simulink model "STM32_UART_PWM_OUTPUT"  (R2024b)
settings: Solver=ode4  StartTime=0.0  StopTime=Tsim  FixedStep=0.005  RelTol=1e-3  EnableMultiTasking=on
values from neighbouring files (symbols this model uses):
  circle_dir = 1    [STM32_UART_PWM_OUTPUT_SETUP.m]
  DEG_TO_RAD_F32 = single(pi / 180.0)    [STM32_UART_PWM_OUTPUT_SETUP.m]
  delta_corr_max_rad = single(deg2rad(8.0))    [STM32_UART_PWM_OUTPUT_SETUP.m]
  delta_max_rad = deg2rad(25)    [STM32_UART_PWM_OUTPUT_SETUP.m]
  delta_test_rad = deg2rad(14.6)    [STM32_UART_PWM_OUTPUT_SETUP.m]
  Kd_psi_pid = single(0.0)    [STM32_UART_PWM_OUTPUT_SETUP.m]
  Kd_radius_pid = single(0.0)    [STM32_UART_PWM_OUTPUT_SETUP.m]
  Ki_psi_pid = single(0.0)    [STM32_UART_PWM_OUTPUT_SETUP.m]
  Ki_radius_pid = single(0.0)    [STM32_UART_PWM_OUTPUT_SETUP.m]
  Kp_psi_pid = single(1.0)    [STM32_UART_PWM_OUTPUT_SETUP.m]
  Kp_radius_pid = single(0.65)    [STM32_UART_PWM_OUTPUT_SETUP.m]
  L = 0.26    [STM32_UART_PWM_OUTPUT_SETUP.m]
  psi_offset_max_rad = single(deg2rad(18.0))    [STM32_UART_PWM_OUTPUT_SETUP.m]
  R_ref = 1.0    (= 1)    [STM32_UART_PWM_OUTPUT_SETUP.m]
  Ts_base = 0.005    [STM32_UART_PWM_OUTPUT_SETUP.m]
  xc = 0.0    (= 0)    [STM32_UART_PWM_OUTPUT_SETUP.m]
  yc = 0.0    (= 0)    [STM32_UART_PWM_OUTPUT_SETUP.m]
libraries: slpidlib x2, stm32f4xxblockslib x1, stm32blockslib x1
settings Model: STM32="{\"UARTRead\":{\"ID\":\"STM32_UART_PWM_OUTPUT:145\"},\"PWMOutput\":{\"ID\":\"STM32_UART_PWM_OUTPUT:160\"}}"  Creator=mateu  LastModifiedBy=mateu
settings OptimizationCC: DefaultParameterBehavior=Inlined  EnhancedBackFolding=on  PassReuseOutputArgsAs=Individual arguments  ZeroExternalMemoryAtStartup=off  ZeroInternalMemoryAtStartup=off  MaxStackSize=512  OptimizeBlockOrder=speed  DifferentSizesBufferReuse=on  OptimizationCustomize=off  EfficientTunableParamExpr=on
settings DebuggingCC: ParameterTunabilityLossMsg=error
settings HardwareCC: ProdBitPerPointer=32  ProdBitPerSizeT=32  ProdBitPerPtrDiffT=32  ProdLargestAtomicInteger=Long  ProdLargestAtomicFloat=Double  ProdWordSize=32  ProdLongLongMode=on  ProdHWDeviceType=ARM Compatible->ARM Cortex-M
settings SFSimCC: MATLABDynamicMemAlloc=off
settings RTWCC: Description=Embedded Coder  SystemTargetFile=ert.tlc  HardwareBoard=STM32L4xx Based  TemplateMakefile=ert_default_tmf  Toolchain=GNU Tools for ARM Embedded Processors
settings CodeAppCC: ForceParamTrailComments=on  IgnoreCustomStorageClasses=off  OperatorAnnotations=on  SimulinkDataObjDesc=on  SFDataObjDesc=on  InsertBlockDesc=on
settings ERTTargetCC: TargetLangStandard=C99 (ISO)  CodeReplacementLibrary=ARM Cortex-M  ExtModeTransport=3  ExtModeStaticAlloc=on  ExtModeStaticAllocSize=2048  ExtModeMexFile=ext_xcp  ExtModeIntrfLevel=Level2 - Open

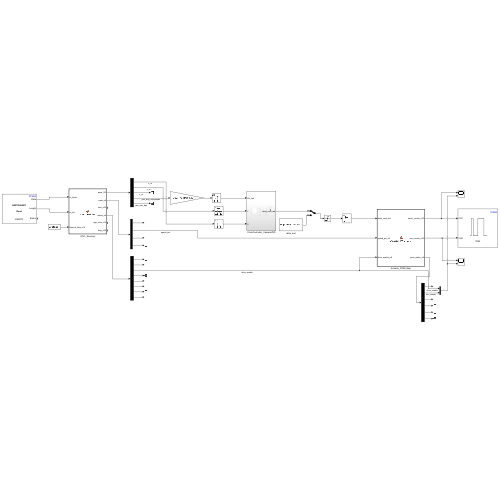
[thumbnail: Simulink's stored preview of the top-level diagram]
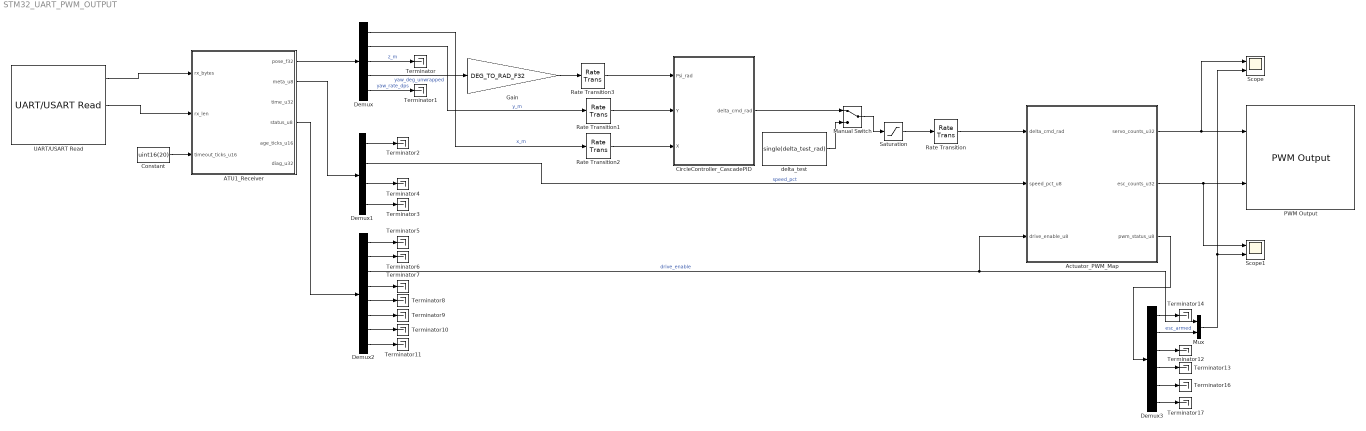
== system STM32_UART_PWM_OUTPUT ==
  ATU1_Receiver : MATLAB Function  TreatAsAtomicUnit=on
  Actuator_PWM_Map : MATLAB Function  TreatAsAtomicUnit=on
  CircleController_CascadePID : Subsystem
  Constant : Constant  Value=uint16(20)
  Demux : Demux  Outputs=5
  Demux1 : Demux
  Demux2 : Demux  Outputs=8
  Demux3 : Demux  Outputs=6
  Gain : Gain  Gain=DEG_TO_RAD_F32
  Manual Switch : ManualSwitch
  Mux : Mux  Inputs=2
  PWM Output : stm32f4xxblockslib/PWM Output  TimerModule=TIM2  DutycycleUnits=Counts  EnableChannel1=on  EnableChannel2=on  EnableChannel3=off  EnableChannel4=off  EnableCounterInput=off  EnableMainOutputInput=off  EnableFrequencyInput=off  SetRCAfterCE=off  OutputDirection=off  OutputMainOutputEnableStatus=off  SampleTime=0.1  EnableSimPort=off  EnableUpdateEvent=off  EnableCaptureCompare1Event=off  EnableCaptureCompare2Event=off  EnableCaptureCompare3Event=off  EnableCaptureCompare4Event=off  EnableTriggerEvent=off  EnableBreakEvent=off  ProcessorFamily=STM32F4  hoistedMaskSrc=ECSoC/ECSimCodegen/PWM Output
  Rate Transition : RateTransition  OutPortSampleTime=Ts_base
  Rate Transition1 : RateTransition  OutPortSampleTime=Ts_control
  Rate Transition2 : RateTransition  OutPortSampleTime=Ts_control
  Rate Transition3 : RateTransition  OutPortSampleTime=Ts_control
  Saturation : Saturate  UpperLimit=delta_max_rad  LowerLimit=-delta_max_rad
  Scope : Scope  NumInputPorts=2
  Scope1 : Scope  NumInputPorts=2
  Terminator{,1..14,16..17} (17 alike) : Terminator
  UART/USART Read : stm32blockslib/UART//USART Read  UARTModule=USART3  DataType=uint8  DataLength=64  BlockingMode=off  BlockingTimeout=0.1  OutputLength=on  OutputStatus=on  SampleTime=Ts_base
      settings: LibrarySourceBlock=stm32f4xxblockslib/UART//USART Read
  delta_test : Constant  Value=single(delta_test_rad)
  wires:
  UART/USART Read/1 -> ATU1_Receiver/1(rx_bytes)
  UART/USART Read/2 -> ATU1_Receiver/2(rx_len)
  Demux/4 -> Gain/1  "yaw_deg_unwrapped"
  Rate Transition1/1 -> CircleController_CascadePID/2(Y)
  Rate Transition2/1 -> CircleController_CascadePID/1(X)
  ATU1_Receiver/1(pose_f32) -> Demux/1
  Demux/1 -> Rate Transition2/1  "x_m"
  Demux/2 -> Rate Transition1/1  "y_m"
  Demux/3 -> Terminator/1  "z_m"
  Demux/5 -> Terminator1/1  "yaw_rate_dps"
  Rate Transition3/1 -> CircleController_CascadePID/3(Psi_rad)
  Gain/1 -> Rate Transition3/1
  CircleController_CascadePID/1(delta_cmd_rad) -> Manual Switch/1
  delta_test/1 -> Manual Switch/2
  Manual Switch/1 -> Saturation/1
  Constant/1 -> ATU1_Receiver/3(timeout_ticks_u16)
  Saturation/1 -> Rate Transition/1
  ATU1_Receiver/2(meta_u8) -> Demux1/1
  Demux1/1 -> Terminator2/1
  Demux1/3 -> Terminator4/1
  Demux1/4 -> Terminator3/1
  ATU1_Receiver/4(status_u8) -> Demux2/1
  Demux2/1 -> Terminator5/1
  Demux2/2 -> Terminator6/1
  Demux2/4 -> Terminator7/1
  Demux2/5 -> Terminator8/1
  Demux2/6 -> Terminator9/1
  Demux2/7 -> Terminator10/1
  Demux2/8 -> Terminator11/1
  Rate Transition/1 -> Actuator_PWM_Map/1(delta_cmd_rad)
  Demux1/2 -> Actuator_PWM_Map/2(speed_pct_u8)  "speed_pct"
  Demux2/3 -> Mux/1, Actuator_PWM_Map/3(drive_enable_u8)  "drive_enable"
  Actuator_PWM_Map/1(servo_counts_u32) -> Scope/1, PWM Output/1
  Actuator_PWM_Map/2(esc_counts_u32) -> Scope1/1, PWM Output/2
  Actuator_PWM_Map/3(pwm_status_u8) -> Demux3/1
  Demux3/1 -> Terminator14/1
  Demux3/2 -> Mux/2  "esc_armed"
  Demux3/3 -> Terminator12/1
  Demux3/4 -> Terminator13/1
  Demux3/5 -> Terminator16/1
  Demux3/6 -> Terminator17/1
  Mux/1 -> Scope/2, Scope1/2

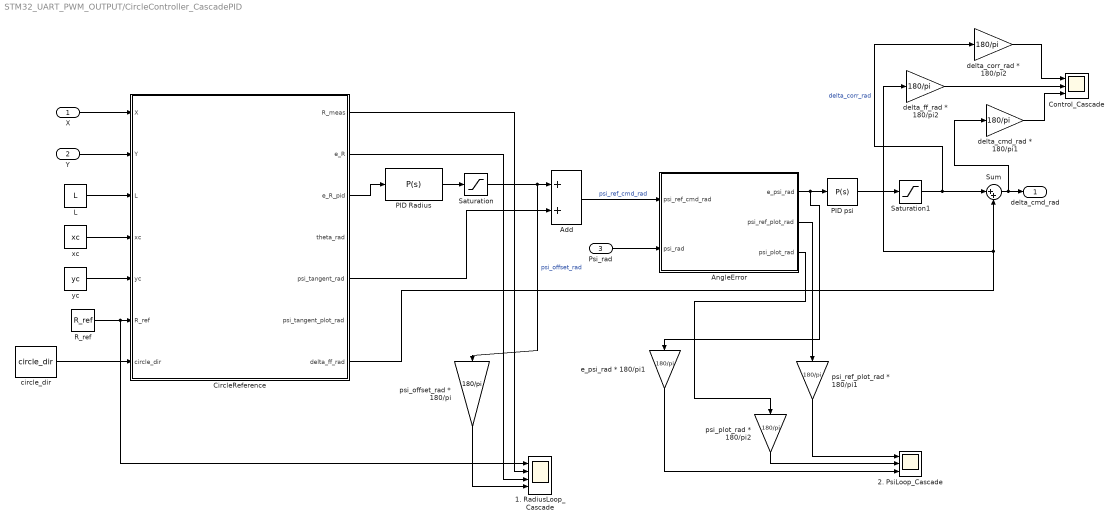
== system STM32_UART_PWM_OUTPUT/CircleController_CascadePID ==
  X : Inport
  Y : Inport  Port=2
  Psi_rad : Inport  Port=3
  1. RadiusLoop_Cascade : Scope  NumInputPorts=4
  2. PsiLoop_Cascade : Scope  NumInputPorts=3
  Add : Sum
  AngleError : MATLAB Function  TreatAsAtomicUnit=on
  CircleReference : MATLAB Function  TreatAsAtomicUnit=on
  Control_Cascade : Scope  NumInputPorts=3
  L : Constant  Value=L
  PID Radius : slpidlib/PID Controller  Controller=P  Form=Parallel  TimeDomain=Continuous-time  UseExternalTs=off  SampleTime=-1  IntegratorMethod=Forward Euler  FilterMethod=Forward Euler  ControllerParametersSource=internal  P=Kp_radius_pid  I=Ki_radius_pid  UseKiTs=off  D=Kd_radius_pid  UseExternalDerivativeSource=off  N=171.856773592637  UseFilter=on  TunerSelectOption=Transfer Function Based (PID Tuner App)  InitialConditionSource=internal  InitialConditionForIntegrator=0  InitialConditionForFilter=0  DifferentiatorICPrevScaledInput=0  ExternalReset=none  TrackingMode=off  Kt=1  LimitOutput=off  SatLimitsSource=internal  UpperSaturationLimit=inf  LowerSaturationLimit=-inf  LinearizeAsGain=on  AntiWindupMode=none  Kb=1  LimitIntegrator=off  UpperIntegratorSaturationLimit=inf  LowerIntegratorSaturationLimit=-inf  POutMin=[]  POutMax=[]  IOutMin=[]  IOutMax=[]  DOutMin=[]  DOutMax=[]  NOutMin=[]  NOutMax=[]  SumOutMin=[]  SumOutMax=[]  SaturationOutMin=[]  SaturationOutMax=[]  PParamMin=[]  PParamMax=[]  IParamMin=[]  IParamMax=[]  DParamMin=[]  DParamMax=[]  NParamMin=[]  NParamMax=[]  KbParamMin=[]  KbParamMax=[]  KtParamMin=[]  KtParamMax=[]  KbOutMin=[]  KbOutMax=[]  KtOutMin=[]  KtOutMax=[]  IntegratorOutMin=[]  IntegratorOutMax=[]  FilterOutMin=[]  FilterOutMax=[]  SumI1OutMin=[]  SumI1OutMax=[]  SumI2OutMin=[]  SumI2OutMax=[]  SumI3OutMin=[]  SumI3OutMax=[]  SumI4OutMin=[]  SumI4OutMax=[]  SumDOutMin=[]  SumDOutMax=[]  DifferentiatorOutMin=[]  DifferentiatorOutMax=[]  FilterDiffOutCoefMin=[]  FilterDiffOutCoefMax=[]  ReciprocalOutMin=[]  ReciprocalOutMax=[]  SumDenOutMin=[]  SumDenOutMax=[]  SumNumOutMin=[]  SumNumOutMax=[]  DivideOutMin=[]  DivideOutMax=[]  UdiffTsProdOutMin=[]  UdiffTsProdOutMax=[]  NTsProdOutMin=[]  NTsProdOutMax=[]  UintegralTsProdOutMin=[]  UintegralTsProdOutMax=[]  UngainTsProdOutMin=[]  UngainTsProdOutMax=[]  ClampingZeroOutDataTypeStr=Inherit: Inherit via back propagation  ClampingZeroOutMin=[]  ClampingZeroOutMax=[]  FilterDenConstantOutDataTypeStr=Inherit: Inherit via back propagation  FilterDenConstantOutMin=[]  FilterDenConstantOutMax=[]  PCopyOutDataTypeStr=Inherit: Inherit via back propagation  PCopyOutMin=[]  PCopyOutMax=[]  NCopyOutDataTypeStr=Inherit: Inherit via back propagation  NCopyOutMin=[]  NCopyOutMax=[]  IntegratorContinuousStateAttributes=''  IntegratorStateMustResolveToSignalObject=off  IntegratorRTWStateStorageClass=Auto  FilterContinuousStateAttributes=''  FilterStateMustResolveToSignalObject=off  FilterRTWStateStorageClass=Auto  ParallelPVariant=InternalParameters  IdealPVariant=Disabled  IVariant=Disabled  DVariant=Disabled  IntegratorVariant=Disabled  SatVariant=Disabled  AWVariant=Disabled  PCopyVariant=Disabled  TRVariant=Disabled  FdbkBlocksVariant=Forward  IdealPFdbkVariant=Disabled  SatFdbkVariant=Disabled  DerivativeFilterVariant=Disabled  NVariant=Disabled  NCopyVariant=Disabled_SignalSpec  FilterICVariant=Disabled  IntegratorICVariant=Disabled  ExternalResetVariant=Disabled  TRSumVariant=Passthrough  SumFdbkVariant=Disabled  SumVariant=Passthrough_P  TsampFilterVariant=InternalTs  TsampNgainVariant=Passthrough  TsampIntegralVariant=Disabled_SignalSpec  ExternalSaturationOutDataTypeStr=Inherit: Same as second input  DerivativeSourceVariant=Disabled  PreIntVariant=InternalPreInt
  PID psi : slpidlib/PID Controller  Controller=P  Form=Parallel  TimeDomain=Continuous-time  UseExternalTs=off  SampleTime=-1  IntegratorMethod=Forward Euler  FilterMethod=Forward Euler  ControllerParametersSource=internal  P=Kp_psi_pid  I=Ki_psi_pid  UseKiTs=off  D=Kd_psi_pid  UseExternalDerivativeSource=off  N=184.215923888363  UseFilter=on  TunerSelectOption=Transfer Function Based (PID Tuner App)  InitialConditionSource=internal  InitialConditionForIntegrator=0  InitialConditionForFilter=0  DifferentiatorICPrevScaledInput=0  ExternalReset=none  TrackingMode=off  Kt=1  LimitOutput=off  SatLimitsSource=internal  UpperSaturationLimit=inf  LowerSaturationLimit=-inf  LinearizeAsGain=on  AntiWindupMode=none  Kb=1  LimitIntegrator=off  UpperIntegratorSaturationLimit=inf  LowerIntegratorSaturationLimit=-inf  POutMin=[]  POutMax=[]  IOutMin=[]  IOutMax=[]  DOutMin=[]  DOutMax=[]  NOutMin=[]  NOutMax=[]  SumOutMin=[]  SumOutMax=[]  SaturationOutMin=[]  SaturationOutMax=[]  PParamMin=[]  PParamMax=[]  IParamMin=[]  IParamMax=[]  DParamMin=[]  DParamMax=[]  NParamMin=[]  NParamMax=[]  KbParamMin=[]  KbParamMax=[]  KtParamMin=[]  KtParamMax=[]  KbOutMin=[]  KbOutMax=[]  KtOutMin=[]  KtOutMax=[]  IntegratorOutMin=[]  IntegratorOutMax=[]  FilterOutMin=[]  FilterOutMax=[]  SumI1OutMin=[]  SumI1OutMax=[]  SumI2OutMin=[]  SumI2OutMax=[]  SumI3OutMin=[]  SumI3OutMax=[]  SumI4OutMin=[]  SumI4OutMax=[]  SumDOutMin=[]  SumDOutMax=[]  DifferentiatorOutMin=[]  DifferentiatorOutMax=[]  FilterDiffOutCoefMin=[]  FilterDiffOutCoefMax=[]  ReciprocalOutMin=[]  ReciprocalOutMax=[]  SumDenOutMin=[]  SumDenOutMax=[]  SumNumOutMin=[]  SumNumOutMax=[]  DivideOutMin=[]  DivideOutMax=[]  UdiffTsProdOutMin=[]  UdiffTsProdOutMax=[]  NTsProdOutMin=[]  NTsProdOutMax=[]  UintegralTsProdOutMin=[]  UintegralTsProdOutMax=[]  UngainTsProdOutMin=[]  UngainTsProdOutMax=[]  ClampingZeroOutDataTypeStr=Inherit: Inherit via back propagation  ClampingZeroOutMin=[]  ClampingZeroOutMax=[]  FilterDenConstantOutDataTypeStr=Inherit: Inherit via back propagation  FilterDenConstantOutMin=[]  FilterDenConstantOutMax=[]  PCopyOutDataTypeStr=Inherit: Inherit via back propagation  PCopyOutMin=[]  PCopyOutMax=[]  NCopyOutDataTypeStr=Inherit: Inherit via back propagation  NCopyOutMin=[]  NCopyOutMax=[]  IntegratorContinuousStateAttributes=''  IntegratorStateMustResolveToSignalObject=off  IntegratorRTWStateStorageClass=Auto  FilterContinuousStateAttributes=''  FilterStateMustResolveToSignalObject=off  FilterRTWStateStorageClass=Auto  ParallelPVariant=InternalParameters  IdealPVariant=Disabled  IVariant=Disabled  DVariant=Disabled  IntegratorVariant=Disabled  SatVariant=Disabled  AWVariant=Disabled  PCopyVariant=Disabled  TRVariant=Disabled  FdbkBlocksVariant=Forward  IdealPFdbkVariant=Disabled  SatFdbkVariant=Disabled  DerivativeFilterVariant=Disabled  NVariant=Disabled  NCopyVariant=Disabled_SignalSpec  FilterICVariant=Disabled  IntegratorICVariant=Disabled  ExternalResetVariant=Disabled  TRSumVariant=Passthrough  SumFdbkVariant=Disabled  SumVariant=Passthrough_P  TsampFilterVariant=InternalTs  TsampNgainVariant=Passthrough  TsampIntegralVariant=Disabled_SignalSpec  ExternalSaturationOutDataTypeStr=Inherit: Same as second input  DerivativeSourceVariant=Disabled  PreIntVariant=InternalPreInt
  R_ref : Constant  Value=R_ref
  Saturation : Saturate  UpperLimit=psi_offset_max_rad  LowerLimit=-psi_offset_max_rad
  Saturation1 : Saturate  UpperLimit=delta_corr_max_rad  LowerLimit=-delta_corr_max_rad
  Sum : Sum  Inputs=|++
  circle_dir : Constant  Value=circle_dir
  delta_cmd_rad * 180/pi1 : Gain  Gain=180/pi
  delta_corr_rad * 180/pi2 : Gain  Gain=180/pi
  delta_ff_rad * 180/pi2 : Gain  Gain=180/pi
  e_psi_rad * 180/pi1 : Gain  Gain=180/pi
  psi_offset_rad * 180/pi : Gain  Gain=180/pi
  psi_plot_rad * 180/pi2 : Gain  Gain=180/pi
  psi_ref_plot_rad * 180/pi1 : Gain  Gain=180/pi
  xc : Constant  Value=xc
  yc : Constant  Value=yc
  delta_cmd_rad : Outport
  wires:
  X/1 -> CircleReference/1(X)
  Y/1 -> CircleReference/2(Y)
  yc/1 -> CircleReference/5(yc)
  R_ref/1 -> 1. RadiusLoop_Cascade/1, CircleReference/6(R_ref)
  circle_dir/1 -> CircleReference/7(circle_dir)
  L/1 -> CircleReference/3(L)
  xc/1 -> CircleReference/4(xc)
  CircleReference/3(e_R_pid) -> PID Radius/1
  PID Radius/1 -> Saturation/1
  Saturation/1 -> psi_offset_rad * 180/pi/1, Add/1  "psi_offset_rad"
  CircleReference/5(psi_tangent_rad) -> Add/2
  Add/1 -> AngleError/1(psi_ref_cmd_rad)  "psi_ref_cmd_rad"
  Psi_rad/1 -> AngleError/2(psi_rad)
  PID psi/1 -> Saturation1/1
  Saturation1/1 -> delta_corr_rad * 180/pi2/1, Sum/1  "delta_corr_rad"
  Sum/1 -> delta_cmd_rad * 180/pi1/1, delta_cmd_rad/1
  CircleReference/7(delta_ff_rad) -> delta_ff_rad * 180/pi2/1, Sum/2
  CircleReference/1(R_meas) -> 1. RadiusLoop_Cascade/2
  CircleReference/2(e_R) -> 1. RadiusLoop_Cascade/3
  psi_offset_rad * 180/pi/1 -> 1. RadiusLoop_Cascade/4
  AngleError/2(psi_ref_plot_rad) -> psi_ref_plot_rad * 180/pi1/1
  psi_ref_plot_rad * 180/pi1/1 -> 2. PsiLoop_Cascade/1
  psi_plot_rad * 180/pi2/1 -> 2. PsiLoop_Cascade/2
  e_psi_rad * 180/pi1/1 -> 2. PsiLoop_Cascade/3
  AngleError/3(psi_plot_rad) -> psi_plot_rad * 180/pi2/1
  delta_corr_rad * 180/pi2/1 -> Control_Cascade/1
  delta_ff_rad * 180/pi2/1 -> Control_Cascade/2
  delta_cmd_rad * 180/pi1/1 -> Control_Cascade/3
  AngleError/1(e_psi_rad) -> e_psi_rad * 180/pi1/1, PID psi/1

== matlab function STM32_UART_PWM_OUTPUT/Actuator_PWM_Map ==
  data: delta_cmd_rad input; servo_counts_u32 output; speed_pct_u8 input; drive_enable_u8 input; esc_counts_u32 output; pwm_status_u8 output
function [servo_counts_u32, esc_counts_u32, pwm_status_u8] = ...
    Actuator_PWM_Map(delta_cmd_rad, speed_pct_u8, drive_enable_u8)
%#codegen
%
% =========================================================
% Actuator_PWM_Map
% =========================================================
%
% Zamienia:
%   delta_cmd_rad  → impuls serwa TIM2_CH1
%   speed_pct      → impuls ESC TIM2_CH2
%
% Konfiguracja TIM2 w CubeMX:
%   timer clock po prescalerze = 1 MHz
%   1 count = 1 us
%   ARR = 19999
%   okres = 20 ms = 50 Hz
%
% Wejścia:
%   delta_cmd_rad    single  - zadany kąt skrętu [rad]
%   speed_pct_u8     uint8   - komenda 0...100%
%   drive_enable_u8  uint8   - zezwolenie STM32
%
% Wyjścia:
%   servo_counts_u32 uint32  - CCR dla TIM2_CH1
%   esc_counts_u32   uint32  - CCR dla TIM2_CH2
%
% pwm_status_u8:
%   1 = wejściowe drive_enable
%   2 = ESC uzbrojony
%   3 = końcowe actuator_enable
%   4 = skręt ograniczony
%   5 = prędkość ograniczona
%   6 = speed_pct po ograniczeniu
% =========================================================

% ---------------------------------------------------------
% Parametry serwa
% ---------------------------------------------------------

SERVO_LEFT_US   = single(1300.0);
SERVO_CENTER_US = single(1500.0);
SERVO_RIGHT_US  = single(1700.0);

% Początkowy bezpieczny zakres skrętu: +/-10 stopni
SERVO_DELTA_MAX_RAD = single(10.0 * pi / 180.0);

% Zmień na -1, jeżeli serwo skręca odwrotnie
SERVO_DIRECTION = single(1.0);

% ---------------------------------------------------------
% Parametry ESC
% ---------------------------------------------------------

ESC_NEUTRAL_US     = single(1500.0);
ESC_FORWARD_MAX_US = single(2000.0);

% Początkowo maksymalnie 10% komendy
SPEED_TEST_MAX_PCT = single(10.0);

% Ts_base = 0.005 s
% 600 kroków * 0.005 s = 3 sekundy neutralnego sygnału
ESC_ARM_TICKS = uint16(600);

% ---------------------------------------------------------
% Stan uzbrajania ESC
% ---------------------------------------------------------

persistent arm_counter_u16

if isempty(arm_counter_u16)
    arm_counter_u16 = uint16(0);
end

if arm_counter_u16 < ESC_ARM_TICKS
    arm_counter_u16 = arm_counter_u16 + uint16(1);
end

esc_armed = arm_counter_u16 >= ESC_ARM_TICKS;

drive_enable = drive_enable_u8 ~= uint8(0);

actuator_enable = ...
    drive_enable && ...
    esc_armed;

% =========================================================
% SERWO
% =========================================================

delta_requested_rad = single(delta_cmd_rad);

delta_limited_rad = min( ...
    max(delta_requested_rad, -SERVO_DELTA_MAX_RAD), ...
    SERVO_DELTA_MAX_RAD);

steering_limited = ...
    delta_requested_rad ~= delta_limited_rad;

delta_servo_rad = ...
    SERVO_DIRECTION * delta_limited_rad;

delta_normalized = ...
    delta_servo_rad / SERVO_DELTA_MAX_RAD;

if delta_normalized >= single(0.0)

    % 0...+1:
    % środek → prawa strona
    servo_pulse_us = ...
        SERVO_CENTER_US + ...
        delta_normalized * ...
        (SERVO_RIGHT_US - SERVO_CENTER_US);

else

    % -1...0:
    % lewa strona → środek
    servo_pulse_us = ...
        SERVO_CENTER_US + ...
        delta_normalized * ...
        (SERVO_CENTER_US - SERVO_LEFT_US);

end

% Bez zezwolenia serwo wraca na środek
if ~actuator_enable
    servo_pulse_us = SERVO_CENTER_US;
end

servo_pulse_us = min( ...
    max(servo_pulse_us, SERVO_LEFT_US), ...
    SERVO_RIGHT_US);

% =========================================================
% ESC
% =========================================================

speed_requested_pct = single(speed_pct_u8);

% Ograniczenie pełnego zakresu wejściowego
speed_requested_pct = min( ...
    max(speed_requested_pct, single(0.0)), ...
    single(100.0));

% Dodatkowe ograniczenie pierwszych testów
speed_limited_pct = min( ...
    speed_requested_pct, ...
    SPEED_TEST_MAX_PCT);

speed_limited = ...
    speed_requested_pct ~= speed_limited_pct;

% 0% → 1500 us
% 100% → 2000 us
% Przy limicie 10% maksymalny impuls wyniesie 1550 us
esc_pulse_us = ...
    ESC_NEUTRAL_US + ...
    (speed_limited_pct / single(100.0)) * ...
    (ESC_FORWARD_MAX_US - ESC_NEUTRAL_US);

% Brak zezwolenia lub uzbrajanie → neutral
if ~actuator_enable
    esc_pulse_us = ESC_NEUTRAL_US;
end

esc_pulse_us = min( ...
    max(esc_pulse_us, ESC_NEUTRAL_US), ...
    ESC_FORWARD_MAX_US);

% =========================================================
% Wyjścia TIM2 CCR
% =========================================================

servo_counts_u32 = uint32(round(servo_pulse_us));
esc_counts_u32   = uint32(round(esc_pulse_us));

pwm_status_u8 = zeros(6, 1, 'uint8');

pwm_status_u8(1) = uint8(drive_enable);
pwm_status_u8(2) = uint8(esc_armed);
pwm_status_u8(3) = uint8(actuator_enable);
pwm_status_u8(4) = uint8(steering_limited);
pwm_status_u8(5) = uint8(speed_limited);
pwm_status_u8(6) = uint8(round(speed_limited_pct));

end

== matlab function STM32_UART_PWM_OUTPUT/ATU1_Receiver ==
  data: rx_bytes input; pose_f32 output; rx_len input; meta_u8 output; time_u32 output; status_u8 output; age_ticks_u16 output; diag_u32 output; timeout_ticks_u16 input
function [pose_f32, meta_u8, time_u32, status_u8, ...
          age_ticks_u16, diag_u32] = ...
    ATU1_Receiver(rx_bytes, rx_len, timeout_ticks_u16)

% =========================================================
% ATU1_Receiver
% =========================================================
%
% Wejścia:
%
%   rx_bytes [64x1] uint8
%       bajty odebrane z UART/USART Read
%
%   rx_len [1x1] uint8
%       rzeczywista liczba nowych bajtów
%
% Wyjścia:
%
%   pose_f32 [5x1] single
%       1 = x_m
%       2 = y_m
%       3 = z_m
%       4 = yaw_deg_unwrapped
%       5 = yaw_rate_dps
%
%   meta_u8 [4x1] uint8
%       1 = flags
%       2 = speed_pct
%       3 = fps_hz
%       4 = source_id
%
%   time_u32 [2x1] uint32
%       1 = seq
%       2 = unity_t_ms
%
%   status_u8 [8x1] uint8
%       1 = new_frame
%       2 = frame_fresh
%       3 = drive_enable
%       4 = pose_valid
%       5 = deadman
%       6 = move_en
%       7 = safe_to_drive
%       8 = hard_stop
%
%   age_ticks_u16
%       liczba kroków modelu od ostatniej poprawnej ramki
%
%   diag_u32 [4x1] uint32
%       1 = frames_ok
%       2 = crc_bad
%       3 = format_bad
%       4 = timeout_count
%
% Ramka ATU1:
%
%   1-2   header A5 5A
%   3     version 1
%   4     source_id
%   5-8   seq uint32 LE
%   9-12  unity_t_ms uint32 LE
%   13    flags
%   14    speed_pct
%   15    fps_hz
%   16    reserved
%   17-20 x_m single LE
%   21-24 y_m single LE
%   25-28 z_m single LE
%   29-32 yaw_deg_unwrapped single LE
%   33-36 yaw_rate_dps single LE
%   37-38 CRC16 CCITT-FALSE LE
%
% =========================================================

persistent frame_buffer
persistent frame_count

persistent last_pose
persistent last_meta
persistent last_time

persistent age_ticks
persistent frame_seen
persistent previous_frame_fresh

persistent frames_ok
persistent crc_bad
persistent format_bad
persistent timeout_count

if isempty(frame_count)

    frame_buffer = zeros(38, 1, 'uint8');
    frame_count = uint8(0);

    last_pose = zeros(5, 1, 'single');
    last_meta = zeros(4, 1, 'uint8');
    last_time = zeros(2, 1, 'uint32');

    age_ticks = uint16(65535);
    frame_seen = false;
    previous_frame_fresh = false;

    frames_ok = uint32(0);
    crc_bad = uint32(0);
    format_bad = uint32(0);
    timeout_count = uint32(0);
end

new_frame = false;

% =========================================================
% Liczenie wieku ostatniej poprawnej ramki
% =========================================================

if frame_seen

    if age_ticks < uint16(65535)
        age_ticks = age_ticks + uint16(1);
    end

end

% Ograniczenie długości do rozmiaru wejścia
number_of_bytes = uint16(rx_len(1));

if number_of_bytes > uint16(64)
    number_of_bytes = uint16(64);
end

% =========================================================
% Parser strumienia UART
% =========================================================

for k = 1:64

    if uint16(k) <= number_of_bytes

        current_byte = rx_bytes(k);

        % -------------------------------------------------
        % Szukanie pierwszego bajtu nagłówka: 0xA5
        % -------------------------------------------------

        if frame_count == uint8(0)

            if current_byte == uint8(165)

                frame_buffer(1) = current_byte;
                frame_count = uint8(1);

            end

        % -------------------------------------------------
        % Szukanie drugiego bajtu nagłówka: 0x5A
        % -------------------------------------------------

        elseif frame_count == uint8(1)

            if current_byte == uint8(90)

                frame_buffer(2) = current_byte;
                frame_count = uint8(2);

            elseif current_byte == uint8(165)

                % Kolejny 0xA5 może być początkiem nagłówka
                frame_buffer(1) = current_byte;
                frame_count = uint8(1);

            else

                frame_count = uint8(0);

            end

        % -------------------------------------------------
        % Zbieranie pozostałych bajtów
        % -------------------------------------------------

        else

            write_index = double(frame_count) + 1.0;

            frame_buffer(write_index) = current_byte;
            frame_count = frame_count + uint8(1);

            % ---------------------------------------------
            % Odebrano kompletne 38 bajtów
            % ---------------------------------------------

            if frame_count == uint8(38)

                header_ok = ...
                    frame_buffer(1) == uint8(165) && ...
                    frame_buffer(2) == uint8(90);

                version_ok = ...
                    frame_buffer(3) == uint8(1);

                received_crc = bitor( ...
                    uint16(frame_buffer(37)), ...
                    bitshift(uint16(frame_buffer(38)), 8) ...
                );

                calculated_crc = ...
                    crc16_ccitt_false_36bytes(frame_buffer);

                if header_ok && version_ok && ...
                        received_crc == calculated_crc

                    % -------------------------------------
                    % Meta
                    % -------------------------------------

                    last_meta(1) = frame_buffer(13); % flags
                    last_meta(2) = frame_buffer(14); % speed
                    last_meta(3) = frame_buffer(15); % fps
                    last_meta(4) = frame_buffer(4);  % source

                    % -------------------------------------
                    % Czasy
                    % -------------------------------------

                    last_time(1) = ...
                        read_u32_le(frame_buffer, 5);

                    last_time(2) = ...
                        read_u32_le(frame_buffer, 9);

                    % -------------------------------------
                    % Pozycja
                    % -------------------------------------

                    last_pose(1) = ...
                        read_f32_le(frame_buffer, 17);

                    last_pose(2) = ...
                        read_f32_le(frame_buffer, 21);

                    last_pose(3) = ...
                        read_f32_le(frame_buffer, 25);

                    last_pose(4) = ...
                        read_f32_le(frame_buffer, 29);

                    last_pose(5) = ...
                        read_f32_le(frame_buffer, 33);

                    frames_ok = frames_ok + uint32(1);

                    new_frame = true;
                    frame_seen = true;
                    age_ticks = uint16(0);

                elseif ~header_ok || ~version_ok

                    format_bad = format_bad + uint32(1);

                else

                    crc_bad = crc_bad + uint32(1);

                end

                % Po każdej kompletnej ramce wracamy
                % do szukania nowego nagłówka
                frame_count = uint8(0);

            end
        end
    end
end

% =========================================================
% Dekodowanie flag ostatniej poprawnej ramki
% =========================================================

flags = last_meta(1);

pose_valid = ...
    bitand(flags, uint8(1)) ~= 0;

deadman = ...
    bitand(flags, uint8(2)) ~= 0;

move_en = ...
    bitand(flags, uint8(4)) ~= 0;

data_ok = ...
    bitand(flags, uint8(8)) ~= 0;

safe_to_drive = ...
    bitand(flags, uint8(16)) ~= 0;

hard_stop = ...
    bitand(flags, uint8(128)) ~= 0;

frame_fresh = ...
    frame_seen && ...
    age_ticks < uint16(timeout_ticks_u16(1));

pose_finite = ...
    isfinite(last_pose(1)) && ...
    isfinite(last_pose(2)) && ...
    isfinite(last_pose(3)) && ...
    isfinite(last_pose(4)) && ...
    isfinite(last_pose(5));

speed_valid = ...
    last_meta(2) <= uint8(100);

drive_enable = ...
    frame_fresh && ...
    pose_valid && ...
    deadman && ...
    move_en && ...
    data_ok && ...
    safe_to_drive && ...
    ~hard_stop && ...
    pose_finite && ...
    speed_valid;

% =========================================================
% Licznik przejść do timeoutu
% =========================================================

if previous_frame_fresh && ~frame_fresh
    timeout_count = timeout_count + uint32(1);
end

previous_frame_fresh = frame_fresh;

% =========================================================
% Wyjścia
% =========================================================

pose_f32 = last_pose;
meta_u8 = last_meta;
time_u32 = last_time;

status_u8 = zeros(8, 1, 'uint8');

status_u8(1) = uint8(new_frame);
status_u8(2) = uint8(frame_fresh);
status_u8(3) = uint8(drive_enable);
status_u8(4) = uint8(pose_valid);
status_u8(5) = uint8(deadman);
status_u8(6) = uint8(move_en);
status_u8(7) = uint8(safe_to_drive);
status_u8(8) = uint8(hard_stop);

age_ticks_u16 = age_ticks;

diag_u32 = zeros(4, 1, 'uint32');

diag_u32(1) = frames_ok;
diag_u32(2) = crc_bad;
diag_u32(3) = format_bad;
diag_u32(4) = timeout_count;

end


function value = read_u32_le(data, start_index)
%#codegen

value = ...
    uint32(data(start_index)) + ...
    bitshift(uint32(data(start_index + 1)), 8) + ...
    bitshift(uint32(data(start_index + 2)), 16) + ...
    bitshift(uint32(data(start_index + 3)), 24);

end


function value = read_f32_le(data, start_index)
%#codegen

raw = ...
    uint32(data(start_index)) + ...
    bitshift(uint32(data(start_index + 1)), 8) + ...
    bitshift(uint32(data(start_index + 2)), 16) + ...
    bitshift(uint32(data(start_index + 3)), 24);

value = typecast(raw, 'single');

end


function crc = crc16_ccitt_false_36bytes(data)
%#codegen

crc = uint16(65535); % 0xFFFF

for i = 1:36

    crc = bitxor( ...
        crc, ...
        bitshift(uint16(data(i)), 8) ...
    );

    for bit_index = 1:8

        if bitand(crc, uint16(32768)) ~= 0

            crc = bitxor( ...
                bitshift(crc, 1), ...
                uint16(4129) ...
            );

        else

            crc = bitshift(crc, 1);

        end
    end
end

end

== matlab function STM32_UART_PWM_OUTPUT/CircleController_CascadePID/CircleReference ==
  data: X input; R_meas output; Y input; L input; xc input; yc input; R_ref input; circle_dir input; e_R output; e_R_pid output; theta_rad output; psi_tangent_rad output; psi_tangent_plot_rad output; delta_ff_rad output
function [R_meas, e_R, e_R_pid, theta_rad, ...
          psi_tangent_rad, psi_tangent_plot_rad, ...
          delta_ff_rad] = ...
    CircleReference(X, Y, L, xc, yc, R_ref, circle_dir)
%#codegen

dx = X - xc;
dy = Y - yc;

R_meas = sqrt(dx * dx + dy * dy);

e_R = R_ref - R_meas;

e_R_pid = -circle_dir * e_R;

theta_rad = atan2(dy, dx);

half_pi_f32 = single(pi / 2.0);

psi_tangent_rad = ...
    theta_rad + circle_dir * half_pi_f32;

psi_tangent_plot_rad = atan2( ...
    sin(psi_tangent_rad), ...
    cos(psi_tangent_rad));

delta_ff_rad = ...
    circle_dir * atan(L / R_ref);

end

== matlab function STM32_UART_PWM_OUTPUT/CircleController_CascadePID/AngleError ==
  data: psi_ref_cmd_rad input; e_psi_rad output; psi_rad input; psi_ref_plot_rad output; psi_plot_rad output
function [e_psi_rad, psi_ref_plot_rad, psi_plot_rad] = AngleError(psi_ref_cmd_rad, psi_rad)
% AngleError
%
% Liczy uchyb orientacji:
%
%   e_psi = psi_ref_cmd - psi
%
% z zawinięciem do -pi..pi, żeby uniknąć skoku np. 179 deg -> -179 deg.
%
% PID nie musi mieć wyjścia w tej samej jednostce co wejście.
% Tutaj:
%
%   e_psi_rad -> PID_Psi -> delta_corr_rad
%
% czyli uchyb orientacji [rad] jest przeliczany przez wzmocnienia PID
% na korektę skrętu kół [rad].
%
% To jest analogiczne do:
%
%   uchyb temperatury [degC] -> PID -> moc grzałki [%]

e_psi_rad = atan2(sin(psi_ref_cmd_rad - psi_rad), cos(psi_ref_cmd_rad - psi_rad));

psi_ref_plot_rad = atan2(sin(psi_ref_cmd_rad), cos(psi_ref_cmd_rad));
psi_plot_rad     = atan2(sin(psi_rad),         cos(psi_rad));

end
